simulink model "Dead_Zone_Dynamic_verif"  (Simulink 7.2)
settings: Solver=ode45  StartTime=0.0  StopTime=10.0  RelTol=1e-3
undefined symbols (not defined in the file): sample
libraries: simulink x1
settings Model: Creator=Romain  LastModifiedBy=Romain
settings OptimizationCC: ExpressionDepthLimit=128
settings DebuggingCC: SolverPrmCheckMsg=none  FcnCallInpInsideContextMsg=Enable All  StateNameClashWarn=none  StrictBusMsg=ErrorLevel1
settings CodeAppCC: CustomSymbolStrType=$N$R$M_T
settings GRTTargetCC: TargetFunctionLibrary=C89/C90 (ANSI)

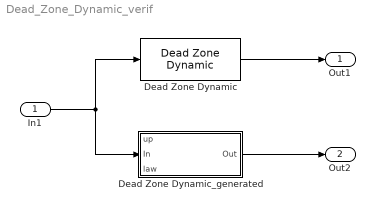
== system Dead_Zone_Dynamic_verif ==
  In1 : Inport  OutDataTypeStr=double  DataType=double
  Dead Zone Dynamic : simulink/Discontinuities/Dead Zone Dynamic
  Dead Zone Dynamic_generated : Subsystem  TreatAsAtomicUnit=on
  Out1 : Outport
  Out2 : Outport  Port=2
  wires:
  In1/1 -> Dead Zone Dynamic_generated/2(In), Dead Zone Dynamic/2
  Dead Zone Dynamic/1 -> Out1/1
  Dead Zone Dynamic_generated/1(Out) -> Out2/1

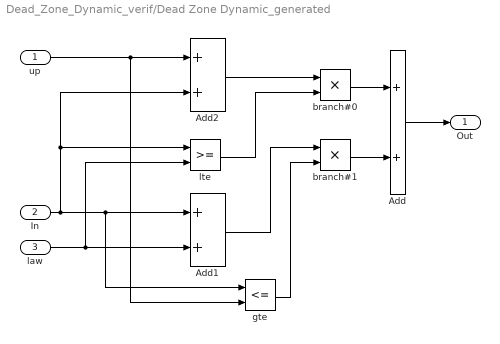
== system Dead_Zone_Dynamic_verif/Dead Zone Dynamic_generated ==
  up : Inport
  In : Inport  Port=2
  law : Inport  Port=3
  Add : Sum
  Add1 : Sum
  Add2 : Sum
  branch#0 : Product  RndMeth=Zero
  branch#1 : Product  RndMeth=Zero
  gte : RelationalOperator  Operator=<=  OutDataTypeStr=boolean  SampleTime=sample  LogicOutDataTypeMode=boolean
  lte : RelationalOperator  OutDataTypeStr=boolean  LogicOutDataTypeMode=boolean
  Out : Outport
  wires:
  In/1 -> Add2/2, lte/1, Add1/1, gte/1
  law/1 -> Add1/2, lte/2
  Add/1 -> Out/1
  up/1 -> Add2/1, gte/2
  Add2/1 -> branch#0/1
  branch#0/1 -> Add/1
  lte/1 -> branch#0/2
  Add1/1 -> branch#1/1
  gte/1 -> branch#1/2
  branch#1/1 -> Add/2
